simulink model "SMC"  (R2025b)
settings: Solver=VariableStepAuto  StartTime=0.0  StopTime=10.0  RelTol=1e-3
InitFcn:
  | run("init.m");
values from neighbouring files (symbols this model uses):
  B = [-1 1 0; 1 0 0; 1 0 1; -1 0 0]    [init.m]    (also in wbr_ctrl.m)
  dq_init = [0;0;0;0]    [init.m]
  q_init = [0;0;0;0]    [init.m]
undefined symbols (not defined in the file or in its folder): K, robot_params
settings Model: Creator=Acer  LastModifiedBy=Acer

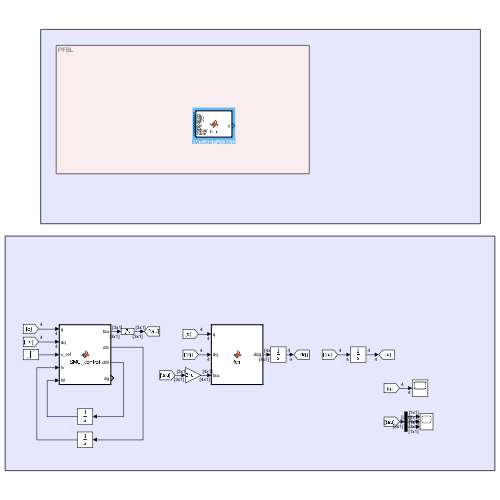
[thumbnail: Simulink's stored preview of the top-level diagram]
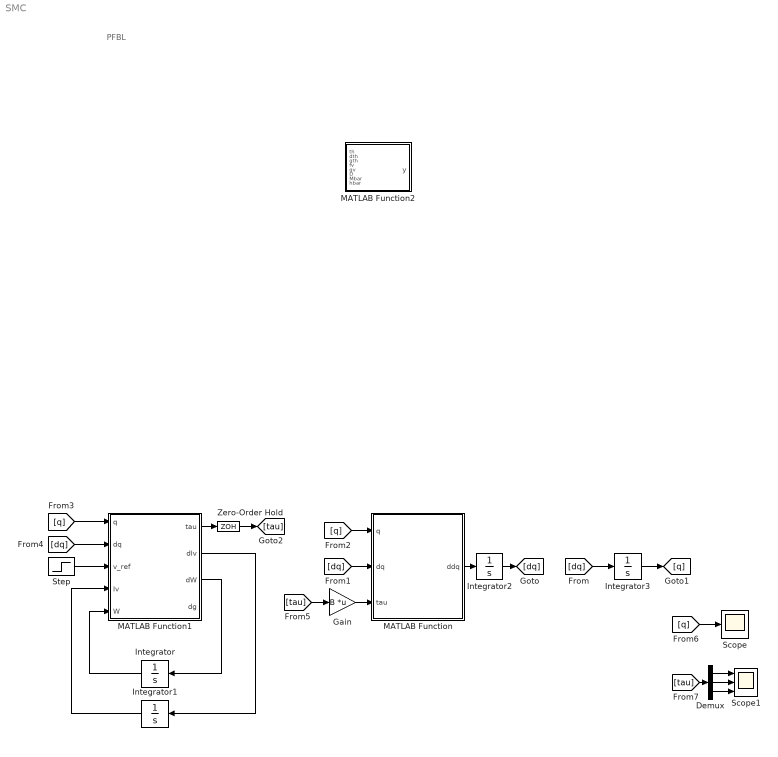
== system SMC ==
  note: PFBL
  Demux : Demux  Outputs=3
  Gain : Gain  Gain=B  Multiplication=Matrix(K*u)
  Integrator : Integrator
  Integrator1 : Integrator
  Integrator2 : Integrator  InitialCondition=dq_init
  Integrator3 : Integrator  InitialCondition=q_init
  MATLAB Function : MATLAB Function  TreatAsAtomicUnit=on
  MATLAB Function1 : MATLAB Function  TreatAsAtomicUnit=on
  MATLAB Function2 : MATLAB Function  TreatAsAtomicUnit=on
  Scope : Scope
      settings: ActiveDisplayYMinimum=-6.2258676593089568  ActiveDisplayYMaximum=47.727726338384315
  Scope1 : Scope  NumInputPorts=3
      settings: ActiveDisplayYMinimum=-22.700835308034456  ActiveDisplayYMaximum=28.535051749705207
  Step : Step  After=0.6  SampleTime=0
  Zero-Order Hold : ZeroOrderHold  SampleTime=1e-2
  wires:
  MATLAB Function1/3(dW) -> Integrator/1
  Integrator/1 -> MATLAB Function1/5(W)
  MATLAB Function1/2(dIv) -> Integrator1/1
  Integrator1/1 -> MATLAB Function1/4(Iv)
  MATLAB Function/1(ddq) -> Integrator2/1
  Integrator2/1 -> [dq]
  [dq] -> Integrator3/1
  Integrator3/1 -> [q]
  [q] -> MATLAB Function/1(q)
  [dq] -> MATLAB Function/2(dq)
  [q] -> MATLAB Function1/1(q)
  [dq] -> MATLAB Function1/2(dq)
  Step/1 -> MATLAB Function1/3(v_ref)
  [q] -> Scope/1
  [tau] -> Gain/1
  Gain/1 -> MATLAB Function/3(tau)
  [tau] -> Demux/1
  Demux/1 -> Scope1/1
  Demux/2 -> Scope1/2
  Demux/3 -> Scope1/3
  MATLAB Function1/1(tau) -> Zero-Order Hold/1
  Zero-Order Hold/1 -> [tau]

== matlab function SMC/MATLAB Function1 ==
  data: q input; tau output; dq input; v_ref input; dIv output; dW output; dg output; Iv input; W input; K parameter; robot_params parameter
function [tau, dIv, dW, dg] = SMC_control(q,      dq,      v_ref, Iv, W, K, robot_params)


[tau, dIv, dW, dg] = wbr_ctrl(q,  dq, v_ref, Iv, W,robot_params, K);

== matlab function SMC/MATLAB Function ==
  data: q input; ddq output; dq input; tau input; B parameter
function ddq = fcn(q,dq, tau, B)

[M,CdQ, Gv] = calc_dynamics(q,dq);

ddq = M\(-CdQ - Gv + tau);

== matlab function SMC/MATLAB Function2 ==
  data: th input; y output; dth input; gth input; fv input; gv input; D input; Mbar input; hbar input
function y = fcn(th, dth, gth, fv, gv, D, Mbar, hbar)
